simulink model "sim02"  (R2020a)
settings: Solver=VariableStepAuto  StartTime=0.0  StopTime=10.0  RelTol=1e-3
values from neighbouring files (symbols this model uses):
  A = [-(Cp*Pp*fp+Ks+Ko)/Cv1,Ko/Cv1;(Cp*Pp*fp+Ko)/Cv2,-(Cp*Pp*fp+Ks+Ko)/Cv2]    [lab01.m]    (also in skrypt.m; sprawozdanie.m)
  B = [(Cp*Pp*fp)/Cv1,Ks/Cv1;0,Ks/Cv2]    [lab01.m]    (also in skrypt.m; sprawozdanie.m)
  C = [1,0;0,1]    [lab01.m]    (also in skrypt.m; sprawozdanie.m)
  czas_skoku = 40    [lab01.m]    (also in sprawozdanie.m = 60)
  D = [0,0;0,0]    [lab01.m]    (also in skrypt.m; sprawozdanie.m)
  duTkz = 0    [lab01.m]    (also in sprawozdanie.m)
  duTzew = 0    [lab01.m]    (also in sprawozdanie.m)
  Tkz = Tab_Tkz(i)    [lab01.m]    (also in skrypt.m; sprawozdanie.m)
  Tzew = Tab_Tzew(i)    [lab01.m]    (also in skrypt.m; sprawozdanie.m)
settings Model: Creator=jakub  LastModifiedBy=jakub

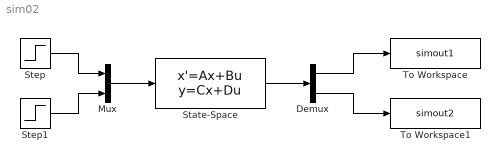
== system sim02 ==
  Demux : Demux  Outputs=2
  Mux : Mux  Inputs=2
  State-Space : StateSpace  A=A  B=B  C=C  D=D  InitialCondition=-A^(-1)*B*u
  Step : Step  Time=czas_skoku  Before=Tkz  After=Tkz+duTkz  SampleTime=0
  Step1 : Step  Time=czas_skoku  Before=Tzew  After=Tzew+duTzew  SampleTime=0
  To Workspace : ToWorkspace  VariableName=simout1  SampleTime=-1
  To Workspace1 : ToWorkspace  VariableName=simout2  SampleTime=-1
  wires:
  Demux/1 -> To Workspace/1
  Step1/1 -> Mux/2
  State-Space/1 -> Demux/1
  Step/1 -> Mux/1
  Demux/2 -> To Workspace1/1
  Mux/1 -> State-Space/1
